simulink model "ex6_2"  (R2024b)
settings: Solver=VariableStepAuto  StartTime=0.0  StopTime=50  RelTol=1e-3
settings Model: Creator=pc  LastModifiedBy=pc

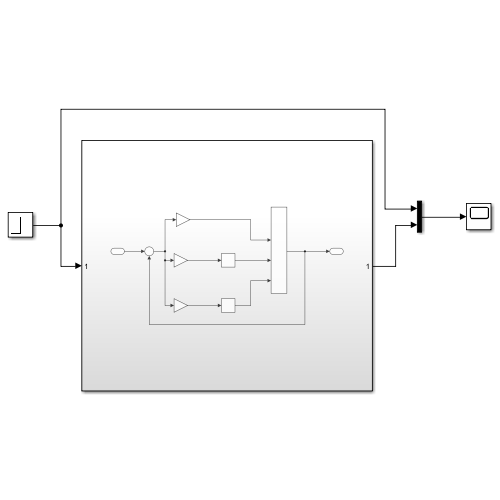
[thumbnail: Simulink's stored preview of the top-level diagram]
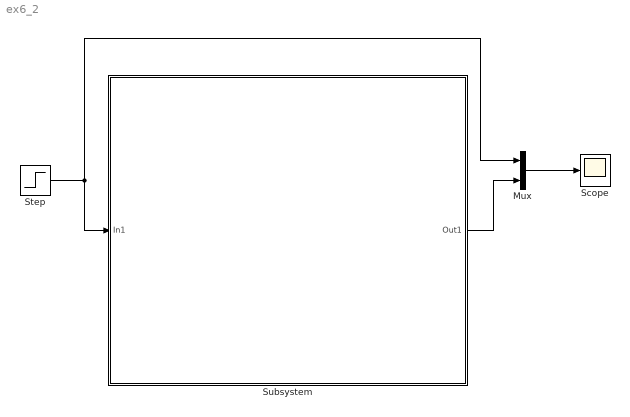
== system ex6_2 ==
  Mux : Mux  Inputs=2
  Scope : Scope
  Step : Step  Time=0  SampleTime=0
  Subsystem : Subsystem
  wires:
  Step/1 -> Subsystem/1(In1), Mux/1
  Mux/1 -> Scope/1
  Subsystem/1(Out1) -> Mux/2

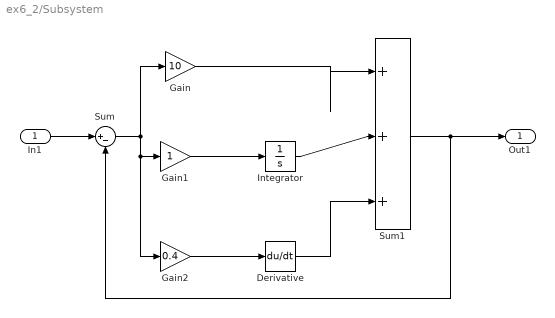
== system ex6_2/Subsystem ==
  In1 : Inport
  Derivative : Derivative
  Gain : Gain  Gain=10
  Gain1 : Gain
  Gain2 : Gain  Gain=0.4
  Integrator : Integrator
  Sum : Sum  Inputs=|+-
  Sum1 : Sum  Inputs=|+++
  Out1 : Outport
  wires:
  Gain2/1 -> Derivative/1
  Gain/1 -> Sum1/1
  In1/1 -> Sum/1
  Sum1/1 -> Out1/1, Sum/2
  Derivative/1 -> Sum1/3
  Sum/1 -> Gain/1, Gain2/1, Gain1/1
  Integrator/1 -> Sum1/2
  Gain1/1 -> Integrator/1
